simulink model "EliminandoBloquedemultiplexacion_90605025"  (R2016a)
settings: Solver=VariableStepAuto  StartTime=0.0  StopTime=420800  RelTol=1e-3
libraries: commutil2 x16, commdigbbndpm3 x16, commchan3 x4
settings Model: Creator=Glynis  LastModifiedBy=Glynis

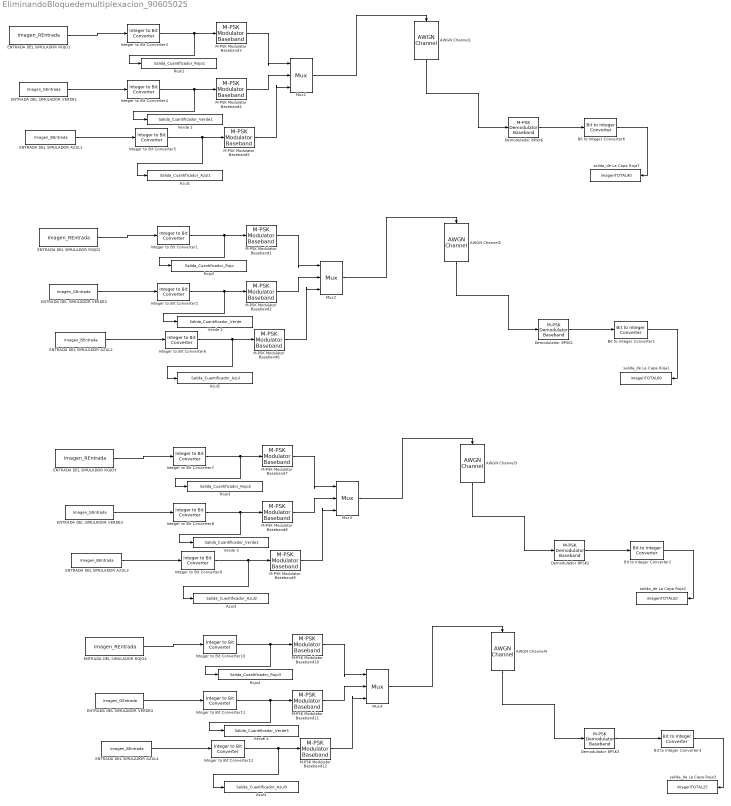
== system EliminandoBloquedemultiplexacion_90605025 ==
  AWGN Channel1 : commchan3/AWGN Channel  InputProcessing=Columns as channels (frame based)  seed=654  noiseMode="Signal to noise ratio  (Eb/No)"  EbNodB=90  EsNodB=10  SNRdB=10  bitsPerSym=8  Ps=1000  Tsym=1  variance=1
  AWGN Channel2 : commchan3/AWGN Channel  InputProcessing=Columns as channels (frame based)  seed=654  noiseMode="Signal to noise ratio  (Eb/No)"  EbNodB=60  EsNodB=10  SNRdB=10  bitsPerSym=8  Ps=1000  Tsym=1  variance=1
  AWGN Channel3 : commchan3/AWGN Channel  InputProcessing=Columns as channels (frame based)  seed=654  noiseMode="Signal to noise ratio  (Eb/No)"  EbNodB=50  EsNodB=10  SNRdB=10  bitsPerSym=8  Ps=1000  Tsym=1  variance=1
  AWGN Channel4 : commchan3/AWGN Channel  InputProcessing=Columns as channels (frame based)  seed=654  noiseMode="Signal to noise ratio  (Eb/No)"  EbNodB=25  EsNodB=10  SNRdB=10  bitsPerSym=8  Ps=1000  Tsym=1  variance=1
  Azul1 : ToWorkspace  VariableName=Salida_Cuantificador_Azul1  SampleTime=-1
      settings: Save2DSignal=2-D array (concatenate along first dimension)
  Azul2 : ToWorkspace  VariableName=Salida_Cuantificador_Azul  SampleTime=-1
      settings: Save2DSignal=2-D array (concatenate along first dimension)
  Azul3 : ToWorkspace  VariableName=Salida_Cuantificador_Azul2  SampleTime=-1
      settings: Save2DSignal=2-D array (concatenate along first dimension)
  Azul4 : ToWorkspace  VariableName=Salida_Cuantificador_Azul3  SampleTime=-1
      settings: Save2DSignal=2-D array (concatenate along first dimension)
  Bit to Integer Converter{1..3,6} (4 alike) : commutil2/Bit to Integer Converter  nbits=8  bitOrder=MSB first  signedOutputValues=Unsigned  outDtype=double  outDtypeSigned=Inherit via internal rule
  Demodulador 8PSK{1..3,6} (4 alike) : commdigbbndpm3/M-PSK Demodulator Baseband  M=8  OutType=Integer  DecType=Hard decision  VarSource=Dialog  Variance=1  Dec=Gray  Mapping=[0:7]  Ph=pi/8  outDtype1=Inherit via internal rule  outDtype2=Inherit via internal rule  derotateFactorWordLen=16  derotateFactorDataTypeStr=Inherit: Same word length as input  derotateFactorLastDataTypeStr=Inherit: Same word length as input
  ENTRADA DEL SIMULADOR AZUL{1..4} (4 alike) : FromWorkspace  VariableName=Imagen_BEntrada  SampleTime=1  OutputAfterFinalValue=Holding final value
  ENTRADA DEL SIMULADOR ROJO{1..4} (4 alike) : FromWorkspace  VariableName=Imagen_REntrada  SampleTime=1  OutputAfterFinalValue=Holding final value
  ENTRADA DEL SIMULADOR VERDE{1..4} (4 alike) : FromWorkspace  VariableName=Imagen_GEntrada  SampleTime=1  OutputAfterFinalValue=Holding final value
  Integer to Bit Converter{1..12} (12 alike) : commutil2/Integer to Bit Converter  nbits=8  signedInputValues=Unsigned  bitOrder=MSB first  outDtype=double
  M-PSK Modulator Baseband{1..12} (12 alike) : commdigbbndpm3/M-PSK Modulator Baseband  M=8  InType=Integer  Enc=Gray  Mapping=[0:7]  Ph=pi/8  outDtype=double  outWordLen=16  outUDDataType=sfix(16)  outFracLenMode=Best precision  outFracLen=15  outDataTypeStr=double  outLastDataTypeStr=double
  Mux{1..4} (4 alike) : Mux  Inputs=3
      settings: DisplayOption=signals
  Rojo1 : ToWorkspace  VariableName=Salida_Cuantificador_Rojo1  SampleTime=-1
      settings: Save2DSignal=2-D array (concatenate along first dimension)
  Rojo2 : ToWorkspace  VariableName=Salida_Cuantificador_Rojo  SampleTime=-1
      settings: Save2DSignal=2-D array (concatenate along first dimension)
  Rojo3 : ToWorkspace  VariableName=Salida_Cuantificador_Rojo2  SampleTime=-1
      settings: Save2DSignal=2-D array (concatenate along first dimension)
  Rojo4 : ToWorkspace  VariableName=Salida_Cuantificador_Rojo3  SampleTime=-1
      settings: Save2DSignal=2-D array (concatenate along first dimension)
  Verde 1 : ToWorkspace  VariableName=Salida_Cuantificador_Verde1  SampleTime=-1
      settings: Save2DSignal=2-D array (concatenate along first dimension)
  Verde 2 : ToWorkspace  VariableName=Salida_Cuantificador_Verde  SampleTime=-1
      settings: Save2DSignal=2-D array (concatenate along first dimension)
  Verde 3 : ToWorkspace  VariableName=Salida_Cuantificador_Verde2  SampleTime=-1
      settings: Save2DSignal=2-D array (concatenate along first dimension)
  Verde 4 : ToWorkspace  VariableName=Salida_Cuantificador_Verde3  SampleTime=-1
      settings: Save2DSignal=2-D array (concatenate along first dimension)
  salida_de La Capa Roja1 : ToWorkspace  VariableName=imagenTOTAL60  SampleTime=1
      settings: Save2DSignal=2-D array (concatenate along first dimension)
  salida_de La Capa Roja2 : ToWorkspace  VariableName=imagenTOTAL50  SampleTime=1
      settings: Save2DSignal=2-D array (concatenate along first dimension)
  salida_de La Capa Roja3 : ToWorkspace  VariableName=imagenTOTAL25  SampleTime=1
      settings: Save2DSignal=2-D array (concatenate along first dimension)
  salida_de La Capa Roja7 : ToWorkspace  VariableName=imagenTOTAL90  SampleTime=1
      settings: Save2DSignal=2-D array (concatenate along first dimension)
  wires:
  Integer to Bit Converter3/1 -> M-PSK Modulator Baseband3/1, Rojo1/1
  ENTRADA DEL SIMULADOR ROJO1/1 -> Integer to Bit Converter3/1
  Mux1/1 -> AWGN Channel1/1
  M-PSK Modulator Baseband3/1 -> Mux1/1
  Integer to Bit Converter4/1 -> M-PSK Modulator Baseband4/1, Verde 1/1
  ENTRADA DEL SIMULADOR VERDE1/1 -> Integer to Bit Converter4/1
  M-PSK Modulator Baseband4/1 -> Mux1/2
  Integer to Bit Converter5/1 -> M-PSK Modulator Baseband5/1, Azul1/1
  ENTRADA DEL SIMULADOR AZUL1/1 -> Integer to Bit Converter5/1
  M-PSK Modulator Baseband5/1 -> Mux1/3
  Demodulador 8PSK6/1 -> Bit to Integer Converter6/1
  AWGN Channel1/1 -> Demodulador 8PSK6/1
  Bit to Integer Converter6/1 -> salida_de La Capa Roja7/1
  Integer to Bit Converter1/1 -> M-PSK Modulator Baseband1/1, Rojo2/1
  ENTRADA DEL SIMULADOR ROJO2/1 -> Integer to Bit Converter1/1
  Mux2/1 -> AWGN Channel2/1
  M-PSK Modulator Baseband1/1 -> Mux2/1
  Integer to Bit Converter2/1 -> M-PSK Modulator Baseband2/1, Verde 2/1
  ENTRADA DEL SIMULADOR VERDE2/1 -> Integer to Bit Converter2/1
  M-PSK Modulator Baseband2/1 -> Mux2/2
  Integer to Bit Converter6/1 -> M-PSK Modulator Baseband6/1, Azul2/1
  ENTRADA DEL SIMULADOR AZUL2/1 -> Integer to Bit Converter6/1
  M-PSK Modulator Baseband6/1 -> Mux2/3
  Demodulador 8PSK1/1 -> Bit to Integer Converter1/1
  AWGN Channel2/1 -> Demodulador 8PSK1/1
  Bit to Integer Converter1/1 -> salida_de La Capa Roja1/1
  Integer to Bit Converter7/1 -> M-PSK Modulator Baseband7/1, Rojo3/1
  ENTRADA DEL SIMULADOR ROJO3/1 -> Integer to Bit Converter7/1
  Mux3/1 -> AWGN Channel3/1
  M-PSK Modulator Baseband7/1 -> Mux3/1
  Integer to Bit Converter8/1 -> M-PSK Modulator Baseband8/1, Verde 3/1
  ENTRADA DEL SIMULADOR VERDE3/1 -> Integer to Bit Converter8/1
  M-PSK Modulator Baseband8/1 -> Mux3/2
  Integer to Bit Converter9/1 -> M-PSK Modulator Baseband9/1, Azul3/1
  ENTRADA DEL SIMULADOR AZUL3/1 -> Integer to Bit Converter9/1
  M-PSK Modulator Baseband9/1 -> Mux3/3
  Demodulador 8PSK2/1 -> Bit to Integer Converter2/1
  AWGN Channel3/1 -> Demodulador 8PSK2/1
  Bit to Integer Converter2/1 -> salida_de La Capa Roja2/1
  Integer to Bit Converter10/1 -> M-PSK Modulator Baseband10/1, Rojo4/1
  ENTRADA DEL SIMULADOR ROJO4/1 -> Integer to Bit Converter10/1
  Mux4/1 -> AWGN Channel4/1
  M-PSK Modulator Baseband10/1 -> Mux4/1
  Integer to Bit Converter11/1 -> M-PSK Modulator Baseband11/1, Verde 4/1
  ENTRADA DEL SIMULADOR VERDE4/1 -> Integer to Bit Converter11/1
  M-PSK Modulator Baseband11/1 -> Mux4/2
  Integer to Bit Converter12/1 -> M-PSK Modulator Baseband12/1, Azul4/1
  ENTRADA DEL SIMULADOR AZUL4/1 -> Integer to Bit Converter12/1
  M-PSK Modulator Baseband12/1 -> Mux4/3
  Demodulador 8PSK3/1 -> Bit to Integer Converter3/1
  AWGN Channel4/1 -> Demodulador 8PSK3/1
  Bit to Integer Converter3/1 -> salida_de La Capa Roja3/1
